simulink model "Phase4_Model_Full_students"  (R2023b)
settings: Solver=FixedStepAuto  StartTime=0.0  StopTime=5  FixedStep=Ts  RelTol=1e-3
values from neighbouring files (symbols this model uses):
  A = [zeros(2,2)  eye(2) ... (first row only)    [Task2_P4.m]    (also in linearized_model_students.m; task1_P4.m; task1_p4.m; task2_P4.m)
  B = [zeros(2,1) ... (first row only)    [Task2_P4.m]    (also in linearized_model_students.m; task1_P4.m; task1_p4.m; task2_P4.m)
  C = [1 0 0 0 ... (first row only)    [Task2_P4.m]    (also in linearized_model_students.m; task1_P4.m; task1_p4.m; task2_P4.m)
  Kf = Kc * T_1    [Task2_P4.m]    (also in linearized_model_students.m; task1_P4.m; task1_p4.m; task2_P4.m)
  L = Lt.'    [Task3_p4.m]    (also in linearized_model_students.m; task3_P4.m)
  Ph = [0.0322261797598 0.0141739364517 0.0605899881507 0.00105505375597 1.7477329169 0.0147577847461]    [ph.mat]
  q10 = 0    [Task2_P4.m]    (also in linearized_model_students.m; task1_P4.m; task1_p4.m; task2_P4.m)
  q20 = pi    (= 3.14159265359)    [Task2_P4.m]    (also in linearized_model_students.m; task1_P4.m; task1_p4.m; task2_P4.m)
  X0 = [0; 0.95*pi; 0; 0]    [Task2_P4.m]    (also in linearized_model_students.m; task1_P4.m; task1_p4.m; task2_P4.m)
settings Model: Creator=shahin  LastModifiedBy=smitj19
settings DataIOCC: ReturnWorkspaceOutputs=off
settings OptimizationCC: ReuseModelBlockBuffer=off

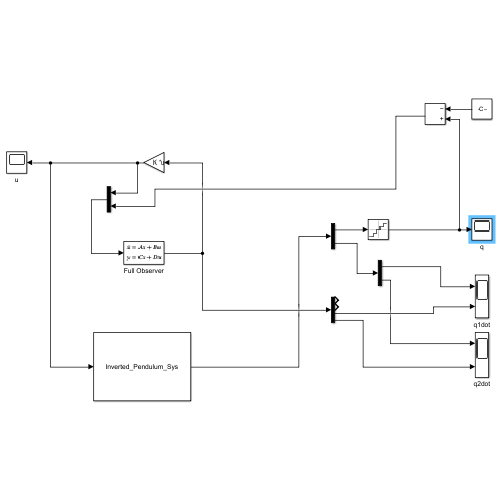
[thumbnail: Simulink's stored preview of the top-level diagram]
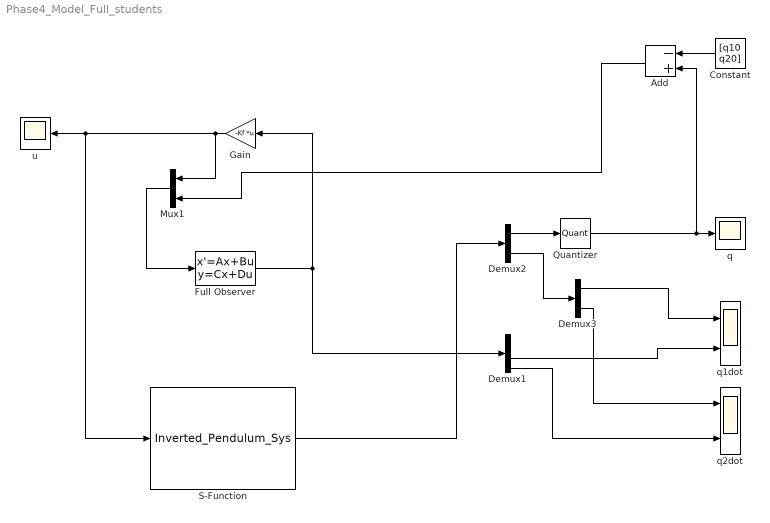
== system Phase4_Model_Full_students ==
  Add : Sum  Inputs=-+
  Constant : Constant  Value="[q10  q20]"
  Demux1 : Demux
  Demux2 : Demux  Outputs=2
  Demux3 : Demux  Outputs=2
  Full Observer : StateSpace  A=A-L*C  B=[B L]  C=eye(4)  D=zeros(4,3)  InitialCondition=[0;0;0;0]
  Gain : Gain  Gain=-Kf  Multiplication=Matrix(K*u)
  Mux1 : Mux  Inputs=2
  Quantizer : Quantizer  QuantizationInterval="[2*pi/2048  2*pi/2048]"
  S-Function : S-Function  FunctionName=Inverted_Pendulum_Sys  Parameters=X0,Ph  SFunctionDeploymentMode=off  EnableBusSupport=off
  q : Scope
  q1dot : Scope  NumInputPorts=2
  q2dot : Scope  NumInputPorts=2
  u : Scope
  wires:
  Demux2/1 -> Quantizer/1
  Add/1 -> Mux1/2
  Quantizer/1 -> Add/2, q/1
  Constant/1 -> Add/1
  Mux1/1 -> Full Observer/1
  Demux2/2 -> Demux3/1
  Demux3/1 -> q1dot/1
  Demux3/2 -> q2dot/1
  Gain/1 -> Mux1/1, S-Function/1, u/1
  Full Observer/1 -> Demux1/1, Gain/1
  Demux1/3 -> q1dot/2
  Demux1/4 -> q2dot/2
  S-Function/1 -> Demux2/1
